simulink model "sampleModel1703"  (R2023a)
settings: Solver=VariableStepAuto  StartTime=0.0  StopTime=10.0  RelTol=1e-3
libraries: hdlsllib x6, simulink x4
settings Model: Creator=user1  LastModifiedBy=user1

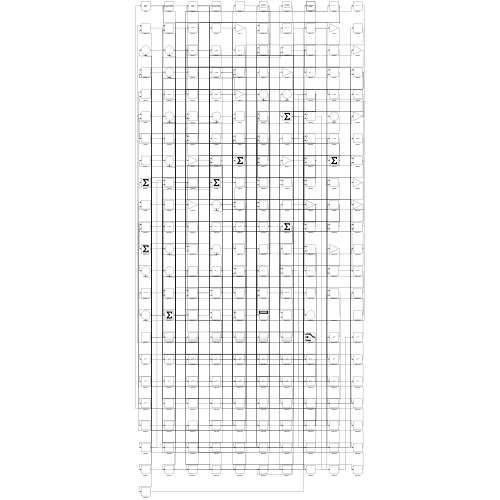
[thumbnail: Simulink's stored preview of the top-level diagram]
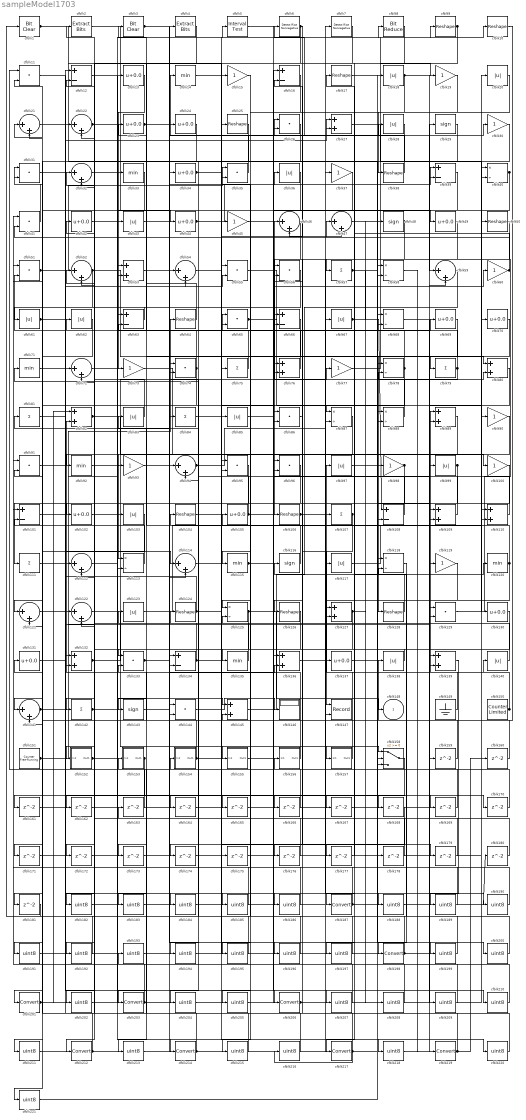
== system sampleModel1703 ==
  cfblk1 : simulink/Logic and Bit Operations/Bit Clear  iBit=0
      settings: LibrarySourceBlock=|
      | hdlsllib/Logic and Bit
      | Operations/Bit Clear
  cfblk{9..10,17,25,38,50,64,104,106,124,126,128} (12 alike) : Reshape
  cfblk{15,19,30,37,45,60,73,77,90,93,98,100,119} (13 alike) : Gain
  cfblk{12,16,39,63,66,101,108,134} (8 alike) : Sum  Inputs=+-
  cfblk{13,23..24,34,42,44,49,69..70,102,105,130..131,137} (14 alike) : Bias  Bias=0.0  SaturateOnIntegerOverflow=off
  cfblk{18,20,28,36,43,61..62,67,83,85,97,99,103,117,123,138,140} (17 alike) : Abs  SaturateOnIntegerOverflow=off
  cfblk{57,75,79,81,84,107,111,142} (8 alike) : Sum  Inputs=+
  cfblk{27,53,76,80,82,89,109..110,127,132,136,139,145} (13 alike) : Sum
  cfblk{11,26,31,35,41,51,55..56,65,74,86,91,95..96,129,133,144} (17 alike) : DotProduct  OutDataTypeStr=Inherit: Inherit via internal rule
  cfblk{21..22,32,46..47,52,54,59,72,94,112,114,121..122,141} (15 alike) : Sum  Inputs=|++
  cfblk{40,58,68,78,87..88,113,118,125} (9 alike) : Product  Inputs=*/  RndMeth=Zero  SaturateOnIntegerOverflow=on
  cfblk{14,33,71,92,115,120,135} (7 alike) : MinMax
  cfblk{29,48,116,143} (4 alike) : Signum
  cfblk146 : Display
  cfblk147 : Record  FileSettingsInternal="{\"entries\":[{\"content\":{\"excelSettings\":{\"content\":{},\"type\":\"Streamout.ExcelSettings\"}},\"type\":\"Streamout.FileSettingStorage\",\"uuid\":\"\"}],\"packageUris\":[\"http:\\/\\/schema.mathworks.com\\/mf0\\/streamout_blocks\\/R2020a\"],\"version\":\"1.0\"}"  Layout=[1 1]  SignalsInternal="{\"entries\":[{\"content\":{\"signals\":[{\"content\":{\"blockPath\":[],\"dimensions\":[1],\"domain\":\"\",\"lineColor\":\"#a2142f\",\"plots\":[1],\"port\":1,\"signalID\":3105,\"signalName\":\"XY Graph:1\"},\"type\":\"RecordBlkView.Signal\",\"uuid\":\"\"},{\"content\":{\"blockPath\":[],\"dimensions\":[1],\"domain\":\"\",\"lineColor\":\"#139fff\",\"plots\":[1],\"port\":2,\"signalID\":3108,\"signalName\":\"XY Graph:2\"},\"type\":\"RecordBlkView.Signal\",\"uuid\":\"\"}]},\"type\":\"RecordBlkView.InputSignals\",\"uuid\":\"\"}],\"packageUris\":[\"http:\\/\\/schema.mathworks.com\\/mf0\\/streamout_blocks\\/R2020a\"],\"version\":\"1.0\"}"  VisualizationBindings="{\"xyplotplugin\":{\"info\":[{\"series\":[{\"bindingParametersList\":[{\"parameter\":\"X-Axis\",\"signalID\":3105,\"signalName\":\"XY Graph:1\"},{\"parameter\":\"Y-Axis\",\"signalID\":3108,\"signalName\":\"XY Graph:2\"}],\"seriesID\":46213}],\"subplotID\":1}]}}"  CompatibilityTag=XY  st=-1
  cfblk149 : Ground
  cfblk150 : hdlsllib/Sources/Counter Limited  uplimit=7  tsamp=-1
  cfblk151 : hdlsllib/Sources/Counter Free-Running  NumBits=16  tsamp=-1
  cfblk152 : Subsystem
      settings: LibrarySourceBlock=|
      | hdlsllib/Ports &
      | Subsystems/Subsystem
  cfblk153 : Subsystem
      settings: LibrarySourceBlock=|
      | hdlsllib/Ports &
      | Subsystems/Subsystem
  cfblk154 : Subsystem
      settings: LibrarySourceBlock=|
      | hdlsllib/Ports &
      | Subsystems/Subsystem
  cfblk155 : Subsystem
      settings: LibrarySourceBlock=|
      | hdlsllib/Ports &
      | Subsystems/Subsystem
  cfblk156 : Subsystem
      settings: LibrarySourceBlock=|
      | hdlsllib/Ports &
      | Subsystems/Subsystem
  cfblk157 : Subsystem
      settings: LibrarySourceBlock=|
      | hdlsllib/Ports &
      | Subsystems/Subsystem
  cfblk158 : Switch  SaturateOnIntegerOverflow=off  InputSameDT=off
  cfblk{159..181} (23 alike) : Delay  SampleTime=1
  cfblk{182..186,188..197,199..200,202,204..205,207..211,213,215..216,218,220..221} (31 alike) : DataTypeConversion  OutDataTypeStr=uint8  SaturateOnIntegerOverflow=off  RndMeth=Floor
  cfblk{187,198,201,203,206,212,214,217,219} (9 alike) : DataTypeConversion  SaturateOnIntegerOverflow=off  RndMeth=Floor
  cfblk2 : simulink/Logic and Bit Operations/Extract Bits  bitsToExtract=Upper half  numBits=8  bitIdxRange=[0 7]  outScalingMode=Preserve fixed-point scaling
      settings: LibrarySourceBlock=|
      | hdlsllib/Logic and Bit
      | Operations/Extract Bits
  cfblk3 : simulink/Logic and Bit Operations/Bit Clear  iBit=0
      settings: LibrarySourceBlock=|
      | hdlsllib/Logic and Bit
      | Operations/Bit Clear
  cfblk4 : simulink/Logic and Bit Operations/Extract Bits  bitsToExtract=Upper half  numBits=8  bitIdxRange=[0 7]  outScalingMode=Preserve fixed-point scaling
      settings: LibrarySourceBlock=|
      | hdlsllib/Logic and Bit
      | Operations/Extract Bits
  cfblk5 : hdlsllib/Logic and Bit Operations/Interval Test  IntervalClosedRight=on  uplimit=0.5  IntervalClosedLeft=on  lowlimit=-0.5  OutDataTypeStr=boolean
  cfblk6 : hdlsllib/Logic and Bit Operations/Detect Rise Nonnegative  vinit=0  OutDataTypeStr=boolean
  cfblk7 : hdlsllib/Logic and Bit Operations/Detect Rise Nonnegative  vinit=0  OutDataTypeStr=boolean
  cfblk8 : hdlsllib/Logic and Bit Operations/Bit Reduce  mode=AND
  cfblk148 : Outport  VectorParamsAs1DForOutWhenUnconnected=off
  wires:
  cfblk41/1 -> cfblk31/1
  cfblk44/1 -> cfblk36/1, cfblk186/1
  cfblk83/1 -> cfblk32/1
  cfblk13/1 -> cfblk73/1
  cfblk69/1 -> cfblk128/1
  cfblk33/1 -> cfblk201/1
  cfblk40/1 -> cfblk43/1, cfblk88/2, cfblk122/2
  cfblk116/1 -> cfblk105/1
  cfblk141/1 -> cfblk64/1, cfblk54/2
  cfblk86/1 -> cfblk26/1
  cfblk113/1 -> cfblk21/1
  cfblk131/1 -> cfblk82/2
  cfblk17/1 -> cfblk19/1
  cfblk105/1 -> cfblk71/1, cfblk207/1
  cfblk132/1 -> cfblk34/1, cfblk22/2
  cfblk59/1 -> cfblk116/1
  cfblk82/1 -> cfblk100/1, cfblk76/2
  cfblk38/1 -> cfblk6/1
  cfblk5/1 -> cfblk79/1
  cfblk67/1 -> cfblk108/1, cfblk48/1
  cfblk56/1 -> cfblk92/1
  cfblk23/1 -> cfblk134/1, cfblk196/1
  cfblk31/1 -> cfblk72/1
  cfblk88/1 -> cfblk46/1
  cfblk122/1 -> cfblk155/1(In1)
  cfblk51/1 -> cfblk35/1, cfblk21/2
  cfblk84/1 -> cfblk15/1
  cfblk109/1 -> cfblk81/1
  cfblk118/1 -> cfblk198/1
  cfblk92/1 -> cfblk113/1
  cfblk157/1(Out1) -> cfblk97/1
  cfblk135/1 -> cfblk52/1
  cfblk1/1 -> cfblk75/1, cfblk25/1
  cfblk70/1 -> cfblk103/1
  cfblk133/1 -> cfblk77/1, cfblk136/2
  cfblk45/1 -> cfblk49/1
  cfblk12/1 -> cfblk214/1
  cfblk52/1 -> cfblk85/1, cfblk121/2
  cfblk153/1(Out1) -> cfblk11/1, cfblk171/1
  cfblk154/1(Out1) -> cfblk62/1, cfblk122/1, cfblk124/1, cfblk167/1, cfblk194/1
  cfblk127/1 -> cfblk208/1, cfblk215/1
  cfblk149/1 -> cfblk89/1
  cfblk129/1 -> cfblk57/1
  cfblk145/1 -> cfblk98/1
  cfblk2/1 -> cfblk94/1
  cfblk61/1 -> cfblk170/1, cfblk211/1
  cfblk77/1 -> cfblk9/1
  cfblk121/1 -> cfblk53/1
  cfblk89/1 -> cfblk102/1
  cfblk10/1 -> cfblk138/1
  cfblk134/1 -> cfblk112/1, cfblk109/1
  cfblk100/1 -> cfblk111/1
  cfblk53/1 -> cfblk144/1
  cfblk9/1 -> cfblk144/2, cfblk213/1
  cfblk156/1(Out1) -> cfblk42/1
  cfblk80/1 -> cfblk89/2
  cfblk124/1 -> cfblk72/2, cfblk158/3
  cfblk103/1 -> cfblk121/1
  cfblk119/1 -> cfblk217/1
  cfblk42/1 -> cfblk44/1
  cfblk21/1 -> cfblk22/1
  cfblk98/1 -> cfblk173/1, cfblk174/1
  cfblk151/1 -> cfblk129/1, cfblk27/2
  cfblk32/1 -> cfblk5/1
  cfblk123/1 -> cfblk70/1
  cfblk46/1 -> cfblk106/1
  cfblk35/1 -> cfblk14/1
  cfblk37/1 -> cfblk142/1
  cfblk73/1 -> cfblk130/1
  cfblk3/1 -> cfblk54/1, cfblk157/1(In1), cfblk114/2
  cfblk64/1 -> cfblk3/1
  cfblk155/1(Out1) -> cfblk99/1
  cfblk14/1 -> cfblk86/1
  cfblk142/1 -> cfblk84/1, cfblk165/1, cfblk166/1, cfblk220/1
  cfblk8/1 -> cfblk87/1
  cfblk108/1 -> cfblk27/1
  cfblk29/1 -> cfblk53/2
  cfblk25/1 -> cfblk63/1
  cfblk125/1 -> cfblk148/1, cfblk183/1
  cfblk72/1 -> cfblk114/1
  cfblk6/1 -> cfblk143/1, cfblk46/2
  cfblk30/1 -> cfblk125/1
  cfblk4/1 -> cfblk212/1
  cfblk79/1 -> cfblk78/2, cfblk2/1, cfblk65/1
  cfblk102/1 -> cfblk69/1
  cfblk18/1 -> cfblk59/1, cfblk40/2, cfblk96/2
  cfblk107/1 -> cfblk147/1, cfblk176/1
  cfblk99/1 -> cfblk115/1, cfblk158/2
  cfblk15/1 -> cfblk135/1
  cfblk150/1 -> cfblk117/1, cfblk140/1
  cfblk55/1 -> cfblk110/2
  cfblk43/1 -> cfblk80/1
  cfblk143/1 -> cfblk30/1
  cfblk115/1 -> cfblk28/1, cfblk168/1
  cfblk22/1 -> cfblk88/1, cfblk145/1
  cfblk57/1 -> cfblk109/2, cfblk178/1
  cfblk81/1 -> cfblk113/2
  cfblk26/1 -> cfblk94/2
  cfblk48/1 -> cfblk127/1, cfblk127/2, cfblk197/1
  cfblk117/1 -> cfblk29/1
  cfblk152/1(Out1) -> cfblk132/1, cfblk188/1
  cfblk66/1 -> cfblk203/1
  cfblk110/1 -> cfblk74/1
  cfblk94/1 -> cfblk67/1, cfblk47/2
  cfblk93/1 -> cfblk39/1
  cfblk34/1 -> cfblk8/1, cfblk199/1
  cfblk140/1 -> cfblk123/1
  cfblk74/1 -> cfblk51/2, cfblk141/1
  cfblk50/1 -> cfblk56/1
  cfblk71/1 -> cfblk55/2
  cfblk137/1 -> cfblk120/1
  cfblk90/1 -> cfblk93/1
  cfblk128/1 -> cfblk107/1
  cfblk85/1 -> cfblk60/1
  cfblk65/1 -> cfblk129/2, cfblk179/1
  cfblk112/1 -> cfblk10/1
  cfblk20/1 -> cfblk187/1
  cfblk96/1 -> cfblk152/1(In1)
  cfblk138/1 -> cfblk137/1
  cfblk106/1 -> cfblk158/1, cfblk76/1
  cfblk19/1 -> cfblk38/1
  cfblk97/1 -> cfblk80/2
  cfblk63/1 -> cfblk61/1
  cfblk49/1 -> cfblk126/1
  cfblk144/1 -> cfblk146/1
  cfblk130/1 -> cfblk133/1
  cfblk75/1 -> cfblk23/1
  cfblk120/1 -> cfblk147/2, cfblk83/1
  cfblk76/1 -> cfblk63/2
  cfblk78/1 -> cfblk17/1, cfblk132/2, cfblk181/1
  cfblk27/1 -> cfblk90/1
  cfblk101/1 -> cfblk206/1
  cfblk58/1 -> cfblk219/1
  cfblk60/1 -> cfblk24/1, cfblk41/2
  cfblk159/1 -> cfblk51/1
  cfblk160/1 -> cfblk133/2
  cfblk36/1 -> cfblk161/1
  cfblk161/1 -> cfblk55/1
  cfblk126/1 -> cfblk162/1
  cfblk162/1 -> cfblk78/1
  cfblk163/1 -> cfblk31/2
  cfblk87/1 -> cfblk164/1
  cfblk164/1 -> cfblk108/2
  cfblk165/1 -> cfblk125/2
  cfblk166/1 -> cfblk74/2
  cfblk167/1 -> cfblk39/2
  cfblk111/1 -> cfblk169/1
  cfblk169/1 -> cfblk26/2
  cfblk170/1 -> cfblk52/2
  cfblk158/1 -> cfblk172/1
  cfblk172/1 -> cfblk59/2
  cfblk173/1 -> cfblk134/2
  cfblk174/1 -> cfblk86/2
  cfblk54/1 -> cfblk175/1
  cfblk175/1 -> cfblk110/1
  cfblk176/1 -> cfblk35/2
  cfblk104/1 -> cfblk177/1
  cfblk177/1 -> cfblk47/1
  cfblk178/1 -> cfblk32/2
  cfblk179/1 -> cfblk112/2
  cfblk180/1 -> cfblk96/1
  cfblk181/1 -> cfblk1/1
  cfblk7/1 -> cfblk182/1
  cfblk182/1 -> cfblk13/1
  cfblk183/1 -> cfblk7/1
  cfblk91/1 -> cfblk184/1
  cfblk184/1 -> cfblk45/1
  cfblk11/1 -> cfblk185/1
  cfblk185/1 -> cfblk91/1
  cfblk186/1 -> cfblk91/2
  cfblk187/1 -> cfblk180/1, cfblk136/1
  cfblk188/1 -> cfblk20/1
  cfblk139/1 -> cfblk189/1
  cfblk189/1 -> cfblk154/1(In1)
  cfblk136/1 -> cfblk190/1
  cfblk190/1 -> cfblk139/1
  cfblk24/1 -> cfblk191/1
  cfblk191/1 -> cfblk139/2
  cfblk95/1 -> cfblk192/1
  cfblk192/1 -> cfblk41/1
  cfblk193/1 -> cfblk95/1
  cfblk194/1 -> cfblk95/2
  cfblk16/1 -> cfblk195/1
  cfblk195/1 -> cfblk131/1
  cfblk196/1 -> cfblk16/1
  cfblk197/1 -> cfblk16/2
  cfblk198/1 -> cfblk145/2, cfblk65/2, cfblk104/1
  cfblk199/1 -> cfblk118/1
  cfblk47/1 -> cfblk200/1
  cfblk200/1 -> cfblk118/2
  cfblk201/1 -> cfblk50/1, cfblk82/1
  cfblk28/1 -> cfblk202/1
  cfblk202/1 -> cfblk33/1
  cfblk203/1 -> cfblk159/1, cfblk141/2, cfblk37/1
  cfblk168/1 -> cfblk204/1
  cfblk204/1 -> cfblk66/1
  cfblk39/1 -> cfblk205/1
  cfblk205/1 -> cfblk66/2
  cfblk206/1 -> cfblk56/2, cfblk40/1
  cfblk207/1 -> cfblk101/1
  cfblk208/1 -> cfblk101/2
  cfblk68/1 -> cfblk209/1
  cfblk209/1 -> cfblk153/1(In1)
  cfblk171/1 -> cfblk210/1
  cfblk210/1 -> cfblk68/1
  cfblk211/1 -> cfblk68/2
  cfblk212/1 -> cfblk11/2, cfblk18/1
  cfblk213/1 -> cfblk4/1
  cfblk214/1 -> cfblk163/1, cfblk87/2
  cfblk215/1 -> cfblk12/1
  cfblk216/1 -> cfblk12/2
  cfblk217/1 -> cfblk216/1, cfblk156/1(In1)
  cfblk114/1 -> cfblk218/1
  cfblk218/1 -> cfblk119/1
  cfblk219/1 -> cfblk193/1, cfblk160/1
  cfblk220/1 -> cfblk58/1
  cfblk62/1 -> cfblk221/1
  cfblk221/1 -> cfblk58/2

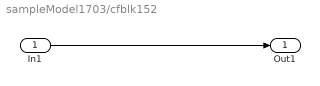
== system sampleModel1703/cfblk152 ==
  In1 : Inport
  Out1 : Outport
  wires:
  In1/1 -> Out1/1

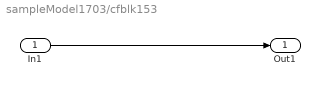
== system sampleModel1703/cfblk153 ==
  In1 : Inport
  Out1 : Outport
  wires:
  In1/1 -> Out1/1

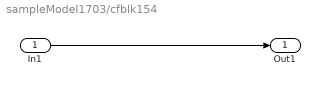
== system sampleModel1703/cfblk154 ==
  In1 : Inport
  Out1 : Outport
  wires:
  In1/1 -> Out1/1

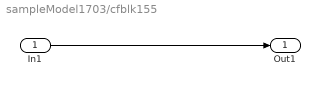
== system sampleModel1703/cfblk155 ==
  In1 : Inport
  Out1 : Outport
  wires:
  In1/1 -> Out1/1

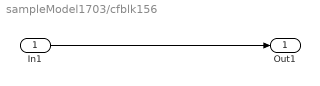
== system sampleModel1703/cfblk156 ==
  In1 : Inport
  Out1 : Outport
  wires:
  In1/1 -> Out1/1

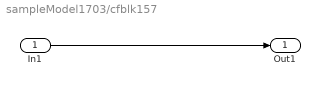
== system sampleModel1703/cfblk157 ==
  In1 : Inport
  Out1 : Outport
  wires:
  In1/1 -> Out1/1
